simulink model "cascade_frequency"  (R2019b)
settings: Solver=VariableStepAuto  StartTime=0.0  StopTime=10.0  RelTol=1e-3
settings Model: Creator=davis  LastModifiedBy=davis

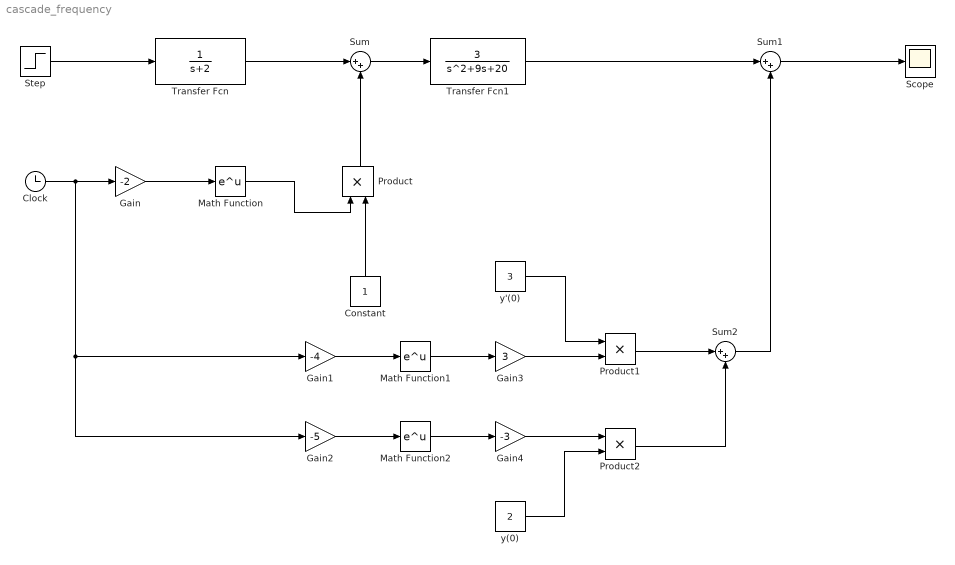
== system cascade_frequency ==
  " y'(0)" : Constant  Value=3
  " y(0)" : Constant  Value=2
  Clock : Clock
  Constant : Constant
  Gain : Gain  Gain=-2
  Gain1 : Gain  Gain=-4
  Gain2 : Gain  Gain=-5
  Gain3 : Gain  Gain=3
  Gain4 : Gain  Gain=-3
  Math Function : Math  SignedPower=off  SaturateOnIntegerOverflow=on
  Math Function1 : Math  SignedPower=off  SaturateOnIntegerOverflow=on
  Math Function2 : Math  SignedPower=off  SaturateOnIntegerOverflow=on
  Product : Product
  Product1 : Product
  Product2 : Product
  Scope : Scope
  Step : Step  Time=0  SampleTime=0
  Sum : Sum  Inputs=|++
  Sum1 : Sum  Inputs=|++
  Sum2 : Sum  Inputs=|++
  Transfer Fcn : TransferFcn  Denominator=[1 2]
  Transfer Fcn1 : TransferFcn  Numerator=[3]  Denominator=[1 9 20]
  wires:
  Math Function/1 -> Product/1
  Step/1 -> Transfer Fcn/1
  Constant/1 -> Product/2
  Transfer Fcn/1 -> Sum/1
  Gain/1 -> Math Function/1
  Product/1 -> Sum/2
  Clock/1 -> Gain2/1, Gain1/1, Gain/1
  " y'(0)"/1 -> Product1/1
  Product2/1 -> Sum2/2
  Product1/1 -> Sum2/1
  Gain2/1 -> Math Function2/1
  Sum1/1 -> Scope/1
  Math Function1/1 -> Gain3/1
  Math Function2/1 -> Gain4/1
  Transfer Fcn1/1 -> Sum1/1
  Sum2/1 -> Sum1/2
  Gain3/1 -> Product1/2
  " y(0)"/1 -> Product2/2
  Sum/1 -> Transfer Fcn1/1
  Gain1/1 -> Math Function1/1
  Gain4/1 -> Product2/1
